simulink model "week2_assignment_ccpid"  (R2020b)
settings: Solver=VariableStepAuto  StartTime=0.0  StopTime=250  FixedStep=0.1  RelTol=1e-3
InitFcn:
  | week2_cruise_control
StopFcn:
  | post_simulation_plots
undefined symbols (not defined in the file or in its folder): distance_travel, Kd, Ki, Kp, m, speed_limit, v_set_speed
libraries: pid_lib x1, simulink x1
settings Model: Creator=anime  LastModifiedBy=anime

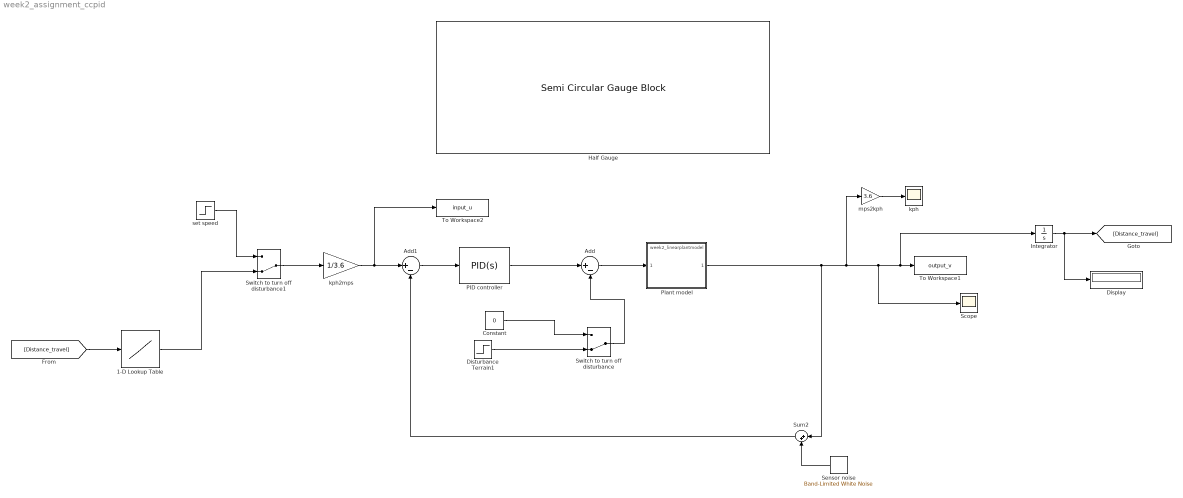
== system week2_assignment_ccpid ==
  1-D Lookup Table : Lookup_n-D  NumberOfTableDimensions=1  BreakpointsForDimension1=distance_travel  Table=speed_limit  InterpMethod=Flat  InternalRulePriority=Speed  RndMeth=Simplest  InputSameDT=on
  Add : Sum  Inputs=|+-
  Add1 : Sum  Inputs=|+-
  Constant : Constant  Value=0
  Display : Display
  Disturbance Terrain1 : Step  Time=100  After=m*9.81*sin(pi/45)  SampleTime=0
  Half Gauge : SemiCircularGaugeBlock  LabelPosition=Hide  ScaleMax=220  TickInterval=25
  Integrator : Integrator
  PID controller : pid_lib/PID Controller  Controller=PID  Form=Parallel  TimeDomain=Continuous-time  UseExternalTs=off  SampleTime=-1  IntegratorMethod=Forward Euler  FilterMethod=Forward Euler  ControllerParametersSource=internal  P=Kp  I=Ki  D=Kd  UseFilter=on  N=100  TunerSelectOption=Transfer Function Based (PID Tuner App)  InitialConditionSource=internal  InitialConditionForIntegrator=0  InitialConditionForFilter=0  DifferentiatorICPrevScaledInput=0  ExternalReset=none  TrackingMode=off  Kt=1  LimitOutput=off  SatLimitsSource=internal  UpperSaturationLimit=inf  LowerSaturationLimit=-inf  LinearizeAsGain=on  AntiWindupMode=none  Kb=1  POutMin=[]  POutMax=[]  IOutMin=[]  IOutMax=[]  DOutMin=[]  DOutMax=[]  NOutMin=[]  NOutMax=[]  SumOutMin=[]  SumOutMax=[]  SaturationOutMin=[]  SaturationOutMax=[]  PParamMin=[]  PParamMax=[]  IParamMin=[]  IParamMax=[]  DParamMin=[]  DParamMax=[]  NParamMin=[]  NParamMax=[]  KbParamMin=[]  KbParamMax=[]  KtParamMin=[]  KtParamMax=[]  KbOutMin=[]  KbOutMax=[]  KtOutMin=[]  KtOutMax=[]  IntegratorOutMin=[]  IntegratorOutMax=[]  FilterOutMin=[]  FilterOutMax=[]  SumI1OutMin=[]  SumI1OutMax=[]  SumI2OutMin=[]  SumI2OutMax=[]  SumI3OutMin=[]  SumI3OutMax=[]  SumI4OutMin=[]  SumI4OutMax=[]  SumDOutMin=[]  SumDOutMax=[]  DifferentiatorOutMin=[]  DifferentiatorOutMax=[]  FilterDiffOutCoefMin=[]  FilterDiffOutCoefMax=[]  ReciprocalOutMin=[]  ReciprocalOutMax=[]  SumDenOutMin=[]  SumDenOutMax=[]  SumNumOutMin=[]  SumNumOutMax=[]  DivideOutMin=[]  DivideOutMax=[]  UdiffTsProdOutMin=[]  UdiffTsProdOutMax=[]  NTsProdOutMin=[]  NTsProdOutMax=[]  UintegralTsProdOutMin=[]  UintegralTsProdOutMax=[]  UngainTsProdOutMin=[]  UngainTsProdOutMax=[]  IntegratorContinuousStateAttributes=''  IntegratorStateMustResolveToSignalObject=off  IntegratorRTWStateStorageClass=Auto  FilterContinuousStateAttributes=''  FilterStateMustResolveToSignalObject=off  FilterRTWStateStorageClass=Auto  ParallelPVariant=InternalParameters  IdealPVariant=Disabled  IVariant=InternalParameters  DVariant=InternalParameters  IntegratorVariant=Continuous  SatVariant=Disabled  AWVariant=Passthrough  PCopyVariant=Disabled  TRVariant=Disabled  FdbkBlocksVariant=Forward  IdealPFdbkVariant=Disabled  SatFdbkVariant=Disabled  DerivativeFilterVariant=ContFilter  NVariant=InternalParameters  NCopyVariant=Disabled  FilterICVariant=InternalICsFilter  IntegratorICVariant=InternalICs  ExternalResetVariant=Disabled  TRSumVariant=Passthrough  SumFdbkVariant=Disabled  SumVariant=Sum_PID  TsampFilterVariant=InternalTs  TsampNgainVariant=Passthrough  TsampIntegralVariant=Passthrough  ExternalSaturationOutDataTypeStr=Inherit: Same as second input
  Plant model : ModelReference  ModelNameDialog=week2_linearplantmodel.slx  SimulationMode=Normal  ModelReferenceVersion=1.2
  Scope : Scope
  Sensor noise : simulink/Sources/Band-Limited White Noise  Cov=[0.001]  Ts=0.1  seed=[23341]
  Sum2 : Sum  Inputs=|++
  Switch to turn off disturbance : ManualSwitch  CurrentSetting=0
  Switch to turn off disturbance1 : ManualSwitch  CurrentSetting=0
  To Workspace1 : ToWorkspace  VariableName=output_v  SaveFormat=Timeseries  SampleTime=-1
  To Workspace2 : ToWorkspace  VariableName=input_u  SaveFormat=Timeseries  SampleTime=-1
  kph : Scope
  kph2mps : Gain  Gain=1/3.6
  mps2kph : Gain  Gain=3.6
  set speed : Step  After=v_set_speed  SampleTime=0
  wires:
  PID controller/1 -> Add/1
  Add1/1 -> PID controller/1
  Constant/1 -> Switch to turn off disturbance/1
  Switch to turn off disturbance/1 -> Add/2
  Add/1 -> Plant model/1
  Disturbance Terrain1/1 -> Switch to turn off disturbance/2
  mps2kph/1 -> kph/1
  kph2mps/1 -> To Workspace2/1, Add1/1
  Plant model/1 -> Sum2/1, mps2kph/1, Integrator/1, To Workspace1/1, Scope/1
  Sensor noise/1 -> Sum2/2
  Sum2/1 -> Add1/2
  Integrator/1 -> [Distance_travel], Display/1
  Switch to turn off disturbance1/1 -> kph2mps/1
  set speed/1 -> Switch to turn off disturbance1/1
  [Distance_travel] -> 1-D Lookup Table/1
  1-D Lookup Table/1 -> Switch to turn off disturbance1/2
